simulink model "mbd_example_uart"  (R2022b)
settings: Solver=FixedStepDiscrete  StartTime=0.0  StopTime=10.0  RelTol=1e-3  EnableMultiTasking=on
PostLoadFcn:
  | run([bdroot '_init']);
InitFcn:
  | checkModelFolder(true); % Optional
  | run([bdroot '_init']);
values from neighbouring files (symbols this model uses):
  T_s_LED1 = 1/LED1_Hz    (= 0.5)    [mbd_example_uart_init.m]
  T_s_LED2 = 1/LED2_Hz    (= 1)    [mbd_example_uart_init.m]
libraries: MbdLib_Uart x18, MbdLib_Digital x13, MbdLib_Timer x7, MbdLib_Sys x4, MbdLib_Required x1
settings Model: Creator=KenYoshioka  LastModifiedBy=KenYoshioka
settings SolverCC: AutoInsertRateTranBlk=on
settings OptimizationCC: DefaultParameterBehavior=Inlined  DefaultUnderspecifiedDataType=single  EnhancedBackFolding=on  BooleansAsBitfields=on  PassReuseOutputArgsAs=Individual arguments  ZeroExternalMemoryAtStartup=off  ZeroInternalMemoryAtStartup=off  OptimizeBlockOrder=speed  DifferentSizesBufferReuse=on  EfficientTunableParamExpr=on
settings DebuggingCC: ParameterTunabilityLossMsg=error
settings HardwareCC: ProdBitPerPointer=32  ProdBitPerSizeT=32  ProdBitPerPtrDiffT=32  ProdLargestAtomicInteger=Long  ProdLargestAtomicFloat=Double  ProdWordSize=32  ProdHWDeviceType=ARM Compatible->ARM Cortex-M
settings ModelReferenceCC: EnableRefExpFcnMdlSchedulingChecks=on  ModelReferenceNumInstancesAllowed=Single
settings SFSimCC: MATLABDynamicMemAlloc=off
settings RTWCC: Description=MBD Embedded Target STM32 Cortex M4 (real-time)  SystemTargetFile=MBD_STM32_stf.tlc  TemplateMakefile=MBD_STM32.tmf  Toolchain=arm-none-eabi - v10.3
settings CodeAppCC: ForceParamTrailComments=on  IgnoreCustomStorageClasses=off  MaxIdLength=255  OperatorAnnotations=on  SimulinkDataObjDesc=on  SFDataObjDesc=on  InsertBlockDesc=on
settings STFCustomTargetCC: MultiwordLength=256  IncludeMdlTerminateFcn=off  CombineOutputUpdateFcns=on  CombineSignalStateStructs=on  SuppressErrorStatus=on  ERTCustomFileBanners=on  SupportContinuousTime=off  RemoveResetFunc=on  MATLABClassNameForMDSCustomization=Simulink.SoftwareTarget.ERTCustomization  UseToolchainInfoCompliant=on  SystemTargetFile=MBD_STM32_stf.tlc
settings ERTTargetCC: ParMdlRefBuildCompliant=off  CompOptLevelCompliant=off  ConcurrentExecutionCompliant=off  IncludeMdlTerminateFcn=off  CombineSignalStateStructs=on  SuppressErrorStatus=on  SupportNonInlinedSFcns=on  ModelStepFunctionPrototypeControlCompliant=off  CPPClassGenCompliant=off  ExtModeStaticAllocSize=2000  InlinedParameterPlacement=NonHierarchical  ERTCustomFileTemplate=mbd_lib_interface.tlc  MaxLineWidth=110

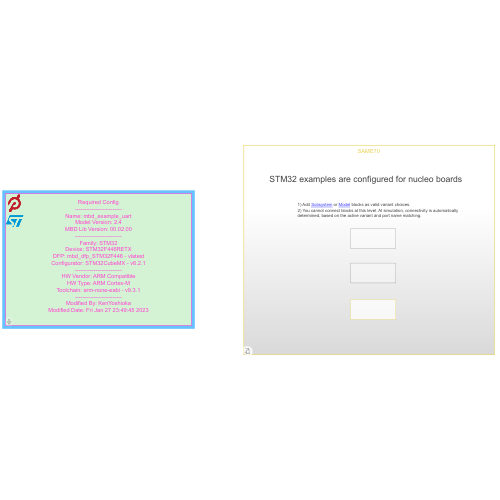
[thumbnail: Simulink's stored preview of the top-level diagram]
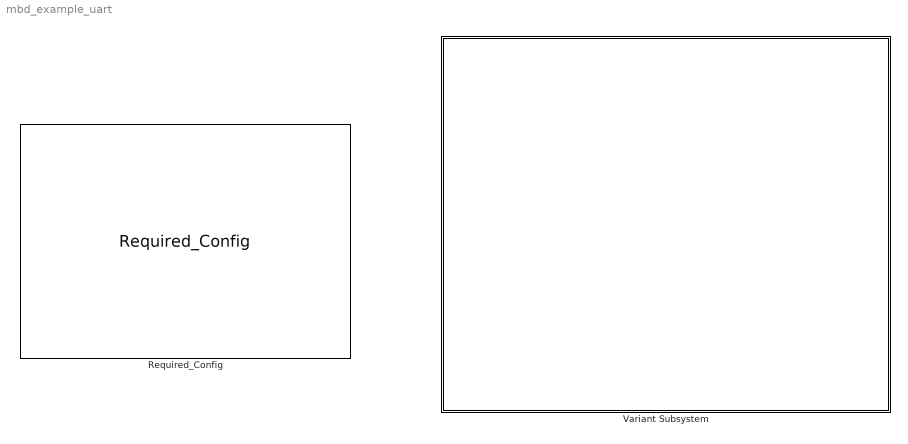
== system mbd_example_uart ==
  Required_Config : MbdLib_Required/Required_Config  Tag=MBD_Target_Info  Param_update=1
      settings: SourceProductName=Peloton Interface Library
  Variant Subsystem : Subsystem  Variant=on

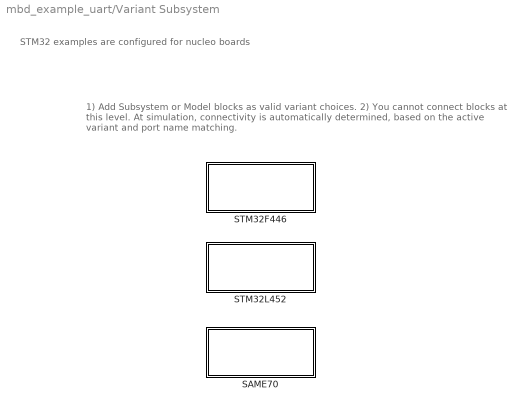
== system mbd_example_uart/Variant Subsystem ==
  note: 1) Add Subsystem or Model blocks as valid variant choices.
      | 2) You cannot connect blocks at this level. At simulation, connectivity is automatically
      | determined, based on the active variant and port name matching.
  note: STM32 examples are configured for nucleo boards
  SAME70 : Subsystem  VariantControl=VAR_MBD_SAME70
  STM32F446 : Subsystem  VariantControl=VAR_MBD_STM32F446
  STM32L452 : Subsystem  VariantControl=VAR_MBD_STM32L452

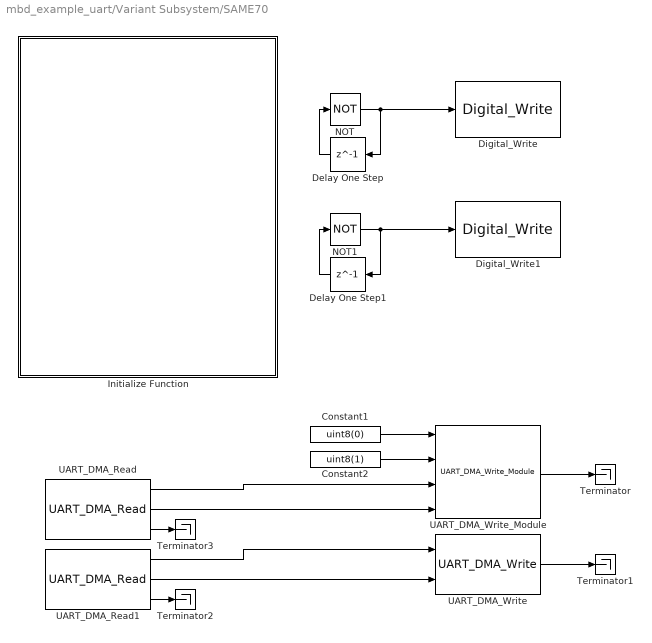
== system mbd_example_uart/Variant Subsystem/SAME70 ==
  Constant1 : Constant  Value=uint8(0)
  Constant2 : Constant  Value=uint8(1)
  Delay One Step : Delay  DelayLength=1  SampleTime=T_s_LED1
  Delay One Step1 : Delay  DelayLength=1  SampleTime=T_s_LED2
  Digital_Write : MbdLib_Digital/Digital_Write  Param_module=D  Param_ch=7  Param_sampleTime=-1
      settings: SourceProductName=Peloton Interface Library
  Digital_Write1 : MbdLib_Digital/Digital_Write  Param_module=D  Param_ch=8  Param_sampleTime=-1
      settings: SourceProductName=Peloton Interface Library
  Initialize Function : Subsystem  TreatAsAtomicUnit=on
  NOT : Logic  Operator=NOT  IconShape=distinctive  AllPortsSameDT=off  OutDataTypeStr=boolean
  NOT1 : Logic  Operator=NOT  IconShape=distinctive  AllPortsSameDT=off  OutDataTypeStr=boolean
  Terminator{,1..3} (4 alike) : Terminator
  UART_DMA_Read : MbdLib_Uart/UART_DMA_Read  Param_module=0  Param_type=USART  Param_readLim=1  Param_sampleTime=T_s_COMM
      settings: SourceProductName=Peloton Interface Library
  UART_DMA_Read1 : MbdLib_Uart/UART_DMA_Read  Param_module=1  Param_type=USART  Param_readLim=1  Param_sampleTime=T_s_COMM
      settings: SourceProductName=Peloton Interface Library
  UART_DMA_Write : MbdLib_Uart/UART_DMA_Write  Param_module=1  Param_type=USART  Param_sampleTime=-1  Sim_status=0
      settings: SourceProductName=Peloton Interface Library
  UART_DMA_Write_Module : MbdLib_Uart/UART_DMA_Write_Module  Param_instanceNum=1  Param_module1=0  Param_type1=USART  Param_module2=0  Param_type2=UART  Param_module3=0  Param_type3=UART  Param_module4=0  Param_type4=UART  Param_sampleTime=-1  Sim_status=0
      settings: SourceProductName=Peloton Interface Library
  wires:
  UART_DMA_Write_Module/1 -> Terminator/1
  UART_DMA_Read/2 -> UART_DMA_Write_Module/4
  UART_DMA_Write/1 -> Terminator1/1
  UART_DMA_Read1/2 -> UART_DMA_Write/2
  Delay One Step1/1 -> NOT1/1
  NOT/1 -> Digital_Write/1, Delay One Step/1
  UART_DMA_Read/1 -> UART_DMA_Write_Module/3
  NOT1/1 -> Digital_Write1/1, Delay One Step1/1
  Constant1/1 -> UART_DMA_Write_Module/1
  Delay One Step/1 -> NOT/1
  UART_DMA_Read1/1 -> UART_DMA_Write/1
  Constant2/1 -> UART_DMA_Write_Module/2
  UART_DMA_Read1/3 -> Terminator2/1
  UART_DMA_Read/3 -> Terminator3/1

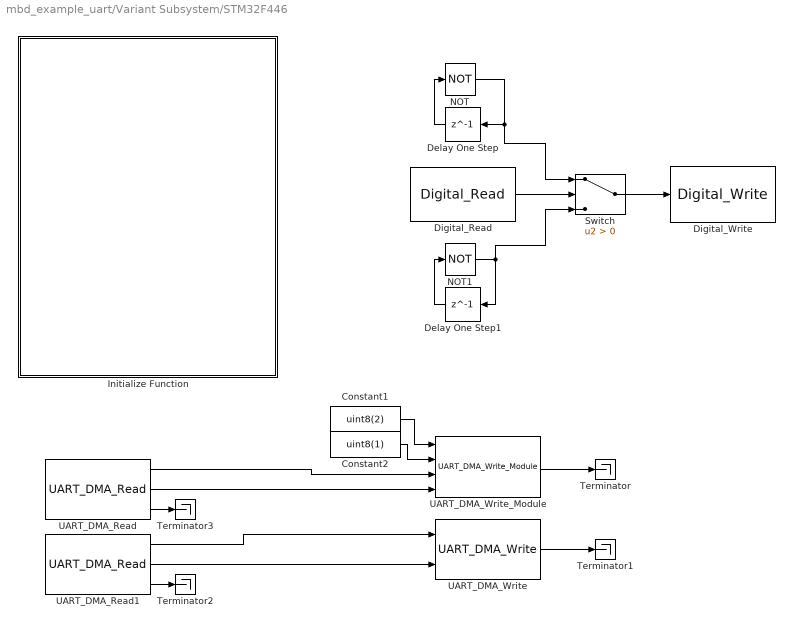
== system mbd_example_uart/Variant Subsystem/STM32F446 ==
  Constant1 : Constant  Value=uint8(2)
  Constant2 : Constant  Value=uint8(1)
  Delay One Step : Delay  DelayLength=1  SampleTime=T_s_LED1
  Delay One Step1 : Delay  DelayLength=1  SampleTime=T_s_LED2
  Digital_Read : MbdLib_Digital/Digital_Read  Param_module=C  Param_ch=13  Param_sampleTime=-1  Sim_invert=off  Sim_out=0
      settings: SourceProductName=Peloton Interface Library
  Digital_Write : MbdLib_Digital/Digital_Write  Param_module=C  Param_ch=10  Param_sampleTime=-1
      settings: SourceProductName=Peloton Interface Library
  Initialize Function : Subsystem  TreatAsAtomicUnit=on
  NOT : Logic  Operator=NOT  IconShape=distinctive  AllPortsSameDT=off  OutDataTypeStr=boolean
  NOT1 : Logic  Operator=NOT  IconShape=distinctive  AllPortsSameDT=off  OutDataTypeStr=boolean
  Switch : Switch  Criteria=u2 > Threshold  SaturateOnIntegerOverflow=off  InputSameDT=off
  Terminator{,1..3} (4 alike) : Terminator
  UART_DMA_Read : MbdLib_Uart/UART_DMA_Read  Param_module=2  Param_type=USART  Param_readLim=1  Param_sampleTime=T_s_COMM
      settings: SourceProductName=Peloton Interface Library
  UART_DMA_Read1 : MbdLib_Uart/UART_DMA_Read  Param_module=3  Param_type=USART  Param_readLim=1  Param_sampleTime=T_s_COMM
      settings: SourceProductName=Peloton Interface Library
  UART_DMA_Write : MbdLib_Uart/UART_DMA_Write  Param_module=3  Param_type=USART  Param_sampleTime=-1  Sim_status=0
      settings: SourceProductName=Peloton Interface Library
  UART_DMA_Write_Module : MbdLib_Uart/UART_DMA_Write_Module  Param_instanceNum=1  Param_module1=1  Param_type1=USART  Param_module2=0  Param_type2=UART  Param_module3=0  Param_type3=UART  Param_module4=0  Param_type4=UART  Param_sampleTime=-1  Sim_status=0
      settings: SourceProductName=Peloton Interface Library
  wires:
  NOT1/1 -> Switch/3, Delay One Step1/1
  NOT/1 -> Switch/1, Delay One Step/1
  Delay One Step/1 -> NOT/1
  Delay One Step1/1 -> NOT1/1
  Digital_Read/1 -> Switch/2
  Switch/1 -> Digital_Write/1
  UART_DMA_Write_Module/1 -> Terminator/1
  UART_DMA_Read/2 -> UART_DMA_Write_Module/4
  UART_DMA_Write/1 -> Terminator1/1
  UART_DMA_Read1/2 -> UART_DMA_Write/2
  UART_DMA_Read/1 -> UART_DMA_Write_Module/3
  Constant1/1 -> UART_DMA_Write_Module/1
  UART_DMA_Read1/1 -> UART_DMA_Write/1
  Constant2/1 -> UART_DMA_Write_Module/2
  UART_DMA_Read1/3 -> Terminator2/1
  UART_DMA_Read/3 -> Terminator3/1

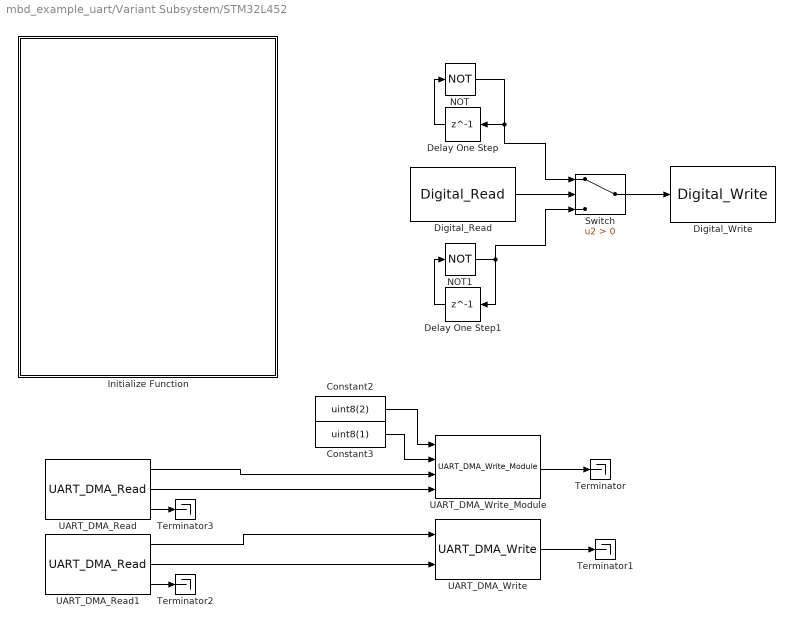
== system mbd_example_uart/Variant Subsystem/STM32L452 ==
  Constant2 : Constant  Value=uint8(2)
  Constant3 : Constant  Value=uint8(1)
  Delay One Step : Delay  DelayLength=1  SampleTime=T_s_LED1
  Delay One Step1 : Delay  DelayLength=1  SampleTime=T_s_LED2
  Digital_Read : MbdLib_Digital/Digital_Read  Param_module=C  Param_ch=13  Param_sampleTime=-1  Sim_invert=off  Sim_out=0
      settings: SourceProductName=Peloton Interface Library
  Digital_Write : MbdLib_Digital/Digital_Write  Param_module=C  Param_ch=10  Param_sampleTime=-1
      settings: SourceProductName=Peloton Interface Library
  Initialize Function : Subsystem  TreatAsAtomicUnit=on
  NOT : Logic  Operator=NOT  IconShape=distinctive  AllPortsSameDT=off  OutDataTypeStr=boolean
  NOT1 : Logic  Operator=NOT  IconShape=distinctive  AllPortsSameDT=off  OutDataTypeStr=boolean
  Switch : Switch  Criteria=u2 > Threshold  SaturateOnIntegerOverflow=off  InputSameDT=off
  Terminator{,1..3} (4 alike) : Terminator
  UART_DMA_Read : MbdLib_Uart/UART_DMA_Read  Param_module=2  Param_type=USART  Param_readLim=1  Param_sampleTime=T_s_COMM
      settings: SourceProductName=Peloton Interface Library
  UART_DMA_Read1 : MbdLib_Uart/UART_DMA_Read  Param_module=3  Param_type=USART  Param_readLim=1  Param_sampleTime=T_s_COMM
      settings: SourceProductName=Peloton Interface Library
  UART_DMA_Write : MbdLib_Uart/UART_DMA_Write  Param_module=3  Param_type=USART  Param_sampleTime=-1  Sim_status=0
      settings: SourceProductName=Peloton Interface Library
  UART_DMA_Write_Module : MbdLib_Uart/UART_DMA_Write_Module  Param_instanceNum=1  Param_module1=1  Param_type1=USART  Param_module2=0  Param_type2=UART  Param_module3=0  Param_type3=UART  Param_module4=0  Param_type4=UART  Param_sampleTime=-1  Sim_status=0
      settings: SourceProductName=Peloton Interface Library
  wires:
  NOT1/1 -> Switch/3, Delay One Step1/1
  NOT/1 -> Switch/1, Delay One Step/1
  Delay One Step/1 -> NOT/1
  Delay One Step1/1 -> NOT1/1
  Digital_Read/1 -> Switch/2
  Switch/1 -> Digital_Write/1
  UART_DMA_Write_Module/1 -> Terminator/1
  UART_DMA_Read/2 -> UART_DMA_Write_Module/4
  UART_DMA_Write/1 -> Terminator1/1
  UART_DMA_Read1/2 -> UART_DMA_Write/2
  UART_DMA_Read/1 -> UART_DMA_Write_Module/3
  UART_DMA_Read1/1 -> UART_DMA_Write/1
  Constant3/1 -> UART_DMA_Write_Module/2
  Constant2/1 -> UART_DMA_Write_Module/1
  UART_DMA_Read1/3 -> Terminator2/1
  UART_DMA_Read/3 -> Terminator3/1

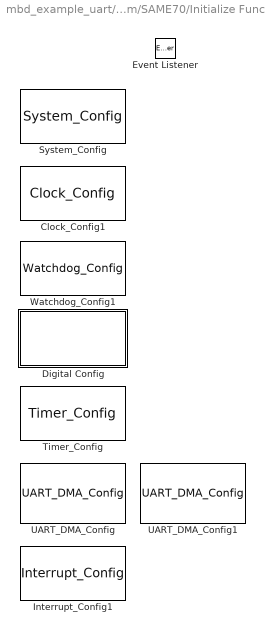
== system mbd_example_uart/Variant Subsystem/SAME70/Initialize Function ==
  Clock_Config1 : MbdLib_Sys/Clock_Config  Priority=10  Param_frequency=Peripheral_Clock_Hz  Param_priority=10  Param_sampleTime=-1
      settings: AttributesFormatString=priority=%<priority>  SourceProductName=Peloton Interface Library
  Digital Config : Subsystem  Priority=30
  Event Listener : EventListener  DisableCoverage=on  EventName=reset
  Interrupt_Config1 : MbdLib_Sys/Interrupt_Config  Priority=120  Param_priority=120  Param_sampleTime=-1
      settings: AttributesFormatString=priority=%<priority>  SourceProductName=Peloton Interface Library
  System_Config : MbdLib_Sys/System_Config  Priority=0  Param_priority=0  Param_sampleTime=-1
      settings: AttributesFormatString=priority=%<priority>  SourceProductName=Peloton Interface Library
  Timer_Config : MbdLib_Timer/Timer_Config  Priority=100  Param_update=1  Param_module=2  Param_step=0  Param_period=Comm_period_cycles  Param_divider=0  Param_step0=0  Param_clksrc0=1  Param_period0=Comm_period_cycles  Param_divider0=0  Param_step1=1  Param_clksrc1=2  Param_period1=LED1_period_cycles  Param_divider1=0  Param_step2=2  Param_clksrc2=2  Param_period2=LED2_period_cycles  Param_divider2=0  Param_priority=100  Param_sampleTime=-1
      settings: AttributesFormatString=priority=%<priority>  SourceProductName=Peloton Interface Library
  UART_DMA_Config : MbdLib_Uart/UART_DMA_Config  Priority=110  Param_module=0  Param_type=USART  Param_speed=921600  Param_dataBits=8  Param_stopBits=0.5  Param_parity=None  Param_priority=110  Param_sampleTime=-1
      settings: AttributesFormatString=priority=%<priority>  SourceProductName=Peloton Interface Library
  UART_DMA_Config1 : MbdLib_Uart/UART_DMA_Config  Priority=110  Param_module=1  Param_type=USART  Param_speed=921600  Param_dataBits=8  Param_stopBits=0.5  Param_parity=None  Param_priority=110  Param_sampleTime=-1
      settings: AttributesFormatString=priority=%<priority>  SourceProductName=Peloton Interface Library
  Watchdog_Config1 : MbdLib_Sys/Watchdog_Config  Priority=20  Param_enable=off  Param_priority=20  Param_sampleTime=-1
      settings: AttributesFormatString=priority=%<priority>  SourceProductName=Peloton Interface Library

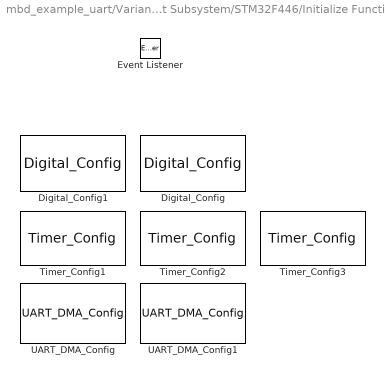
== system mbd_example_uart/Variant Subsystem/STM32F446/Initialize Function ==
  Digital_Config : MbdLib_Digital/Digital_Config  Priority=30  Param_module=C  Param_ch=10  Param_dir=output  Param_pupd=none  Param_default=low  Param_mode=none  Param_drive=low  Param_speed=high  Param_priority=30  Param_sampleTime=-1
      settings: AttributesFormatString=priority=%<priority>  SourceProductName=Peloton Interface Library
  Digital_Config1 : MbdLib_Digital/Digital_Config  Priority=30  Param_module=C  Param_ch=13  Param_dir=input  Param_pupd=pullup  Param_default=low  Param_mode=none  Param_drive=low  Param_speed=high  Param_priority=30  Param_sampleTime=-1
      settings: AttributesFormatString=priority=%<priority>  SourceProductName=Peloton Interface Library
  Event Listener : EventListener  DisableCoverage=on  EventName=reset
  Timer_Config1 : MbdLib_Timer/Timer_Config  Priority=100  Param_update=1  Param_module=1  Param_step=0  Param_period=Comm_period_cycles  Param_divider=Comm_clock_divider  Param_step0=0  Param_clksrc0=0  Param_period0=Comm_period_cycles  Param_divider0=Comm_clock_divider  Param_step1=-1  Param_clksrc1=0  Param_period1=0  Param_divider1=0  Param_step2=-1  Param_clksrc2=0  Param_period2=0  Param_divider2=0  Param_priority=100  Param_sampleTime=-1
      settings: AttributesFormatString=priority=%<priority>  SourceProductName=Peloton Interface Library
  Timer_Config2 : MbdLib_Timer/Timer_Config  Priority=101  Param_update=1  Param_module=6  Param_step=1  Param_period=LED1_period_cycles  Param_divider=LED1_clock_divider  Param_step0=1  Param_clksrc0=0  Param_period0=LED1_period_cycles  Param_divider0=LED1_clock_divider  Param_step1=-1  Param_clksrc1=0  Param_period1=0  Param_divider1=0  Param_step2=-1  Param_clksrc2=0  Param_period2=0  Param_divider2=0  Param_priority=101  Param_sampleTime=-1
      settings: AttributesFormatString=priority=%<priority>  SourceProductName=Peloton Interface Library
  Timer_Config3 : MbdLib_Timer/Timer_Config  Priority=102  Param_update=1  Param_module=7  Param_step=2  Param_period=LED2_period_cycles  Param_divider=LED2_clock_divider  Param_step0=2  Param_clksrc0=0  Param_period0=LED2_period_cycles  Param_divider0=LED2_clock_divider  Param_step1=-1  Param_clksrc1=0  Param_period1=0  Param_divider1=0  Param_step2=-1  Param_clksrc2=0  Param_period2=0  Param_divider2=0  Param_priority=102  Param_sampleTime=-1
      settings: AttributesFormatString=priority=%<priority>  SourceProductName=Peloton Interface Library
  UART_DMA_Config : MbdLib_Uart/UART_DMA_Config  Priority=110  Param_module=2  Param_type=USART  Param_speed=921600  Param_dataBits=8  Param_stopBits=1  Param_parity=None  Param_priority=110  Param_sampleTime=-1
      settings: AttributesFormatString=priority=%<priority>  SourceProductName=Peloton Interface Library
  UART_DMA_Config1 : MbdLib_Uart/UART_DMA_Config  Priority=110  Param_module=3  Param_type=USART  Param_speed=921600  Param_dataBits=8  Param_stopBits=1  Param_parity=None  Param_priority=110  Param_sampleTime=-1
      settings: AttributesFormatString=priority=%<priority>  SourceProductName=Peloton Interface Library

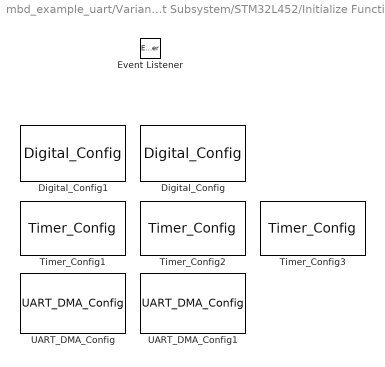
== system mbd_example_uart/Variant Subsystem/STM32L452/Initialize Function ==
  Digital_Config : MbdLib_Digital/Digital_Config  Priority=30  Param_module=C  Param_ch=10  Param_dir=output  Param_pupd=none  Param_default=low  Param_mode=none  Param_drive=low  Param_speed=high  Param_priority=30  Param_sampleTime=-1
      settings: AttributesFormatString=priority=%<priority>  SourceProductName=Peloton Interface Library
  Digital_Config1 : MbdLib_Digital/Digital_Config  Priority=30  Param_module=C  Param_ch=13  Param_dir=input  Param_pupd=pullup  Param_default=low  Param_mode=none  Param_drive=low  Param_speed=high  Param_priority=30  Param_sampleTime=-1
      settings: AttributesFormatString=priority=%<priority>  SourceProductName=Peloton Interface Library
  Event Listener : EventListener  DisableCoverage=on  EventName=reset
  Timer_Config1 : MbdLib_Timer/Timer_Config  Priority=100  Param_update=1  Param_module=6  Param_step=0  Param_period=Comm_period_cycles  Param_divider=Comm_clock_divider  Param_step0=0  Param_clksrc0=0  Param_period0=Comm_period_cycles  Param_divider0=Comm_clock_divider  Param_step1=-1  Param_clksrc1=0  Param_period1=0  Param_divider1=0  Param_step2=-1  Param_clksrc2=0  Param_period2=0  Param_divider2=0  Param_priority=100  Param_sampleTime=-1
      settings: AttributesFormatString=priority=%<priority>  SourceProductName=Peloton Interface Library
  Timer_Config2 : MbdLib_Timer/Timer_Config  Priority=101  Param_update=1  Param_module=15  Param_step=1  Param_period=LED1_period_cycles  Param_divider=LED1_clock_divider  Param_step0=1  Param_clksrc0=0  Param_period0=LED1_period_cycles  Param_divider0=LED1_clock_divider  Param_step1=-1  Param_clksrc1=0  Param_period1=0  Param_divider1=0  Param_step2=-1  Param_clksrc2=0  Param_period2=0  Param_divider2=0  Param_priority=101  Param_sampleTime=-1
      settings: AttributesFormatString=priority=%<priority>  SourceProductName=Peloton Interface Library
  Timer_Config3 : MbdLib_Timer/Timer_Config  Priority=102  Param_update=1  Param_module=16  Param_step=2  Param_period=LED2_period_cycles  Param_divider=LED2_clock_divider  Param_step0=2  Param_clksrc0=0  Param_period0=LED2_period_cycles  Param_divider0=LED2_clock_divider  Param_step1=-1  Param_clksrc1=0  Param_period1=0  Param_divider1=0  Param_step2=-1  Param_clksrc2=0  Param_period2=0  Param_divider2=0  Param_priority=102  Param_sampleTime=-1
      settings: AttributesFormatString=priority=%<priority>  SourceProductName=Peloton Interface Library
  UART_DMA_Config : MbdLib_Uart/UART_DMA_Config  Priority=110  Param_module=2  Param_type=USART  Param_speed=115200  Param_dataBits=8  Param_stopBits=1  Param_parity=None  Param_priority=110  Param_sampleTime=-1
      settings: AttributesFormatString=priority=%<priority>  SourceProductName=Peloton Interface Library
  UART_DMA_Config1 : MbdLib_Uart/UART_DMA_Config  Priority=110  Param_module=3  Param_type=USART  Param_speed=115200  Param_dataBits=8  Param_stopBits=1  Param_parity=None  Param_priority=110  Param_sampleTime=-1
      settings: AttributesFormatString=priority=%<priority>  SourceProductName=Peloton Interface Library

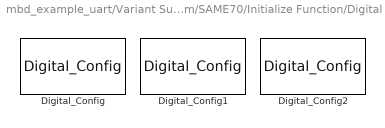
== system mbd_example_uart/Variant Subsystem/SAME70/Initialize Function/Digital Config ==
  Digital_Config : MbdLib_Digital/Digital_Config  Priority=0  Param_module=D  Param_ch=7  Param_dir=output  Param_pupd=none  Param_default=low  Param_mode=none  Param_drive=low  Param_speed=low  Param_priority=0  Param_sampleTime=-1
      settings: SourceProductName=Peloton Interface Library
  Digital_Config1 : MbdLib_Digital/Digital_Config  Priority=0  Param_module=D  Param_ch=8  Param_dir=output  Param_pupd=none  Param_default=low  Param_mode=none  Param_drive=low  Param_speed=low  Param_priority=0  Param_sampleTime=-1
      settings: SourceProductName=Peloton Interface Library
  Digital_Config2 : MbdLib_Digital/Digital_Config  Priority=0  Param_module=D  Param_ch=9  Param_dir=output  Param_pupd=none  Param_default=low  Param_mode=none  Param_drive=low  Param_speed=low  Param_priority=0  Param_sampleTime=-1
      settings: SourceProductName=Peloton Interface Library
